simulink model "cps_fast_network_v2"  (R2012b)
settings: Solver=FixedStepDiscrete  StartTime=0.0  StopTime=8.5  RelTol=20e-5
model workspace (MAT data in the model file):
  ini_block_hpos = -0.4
  ini_block_vpos = 0.11
  ini_nozzle_vpos = 0.3
settings Model: Creator=pmosterm  LastModifiedBy=pmosterm
settings SolverCC: ZcThreshold=2e-5  MaxConsecutiveZCs=20  EnableConcurrentExecution=on  ConcurrentTasks=on  ZeroCrossAlgorithm=Adaptive  SolverResetMethod=Robust
settings DataIOCC: SignalLoggingSaveFormat=ModelDataLogs
settings OptimizationCC: InlineParams=on
settings DebuggingCC: ReadBeforeWriteMsg=DisableAll  WriteAfterWriteMsg=DisableAll  WriteAfterReadMsg=DisableAll  AlgebraicLoopMsg=error  UnderspecifiedInitializationDetection=Simplified  FcnCallInpInsideContextMsg=EnableAllAsWarning  ModelReferenceExtraNoncontSigs=warning
settings ModelReferenceCC: ModelReferenceNumInstancesAllowed=Single
settings GRTTargetCC: CombineOutputUpdateFcns=off  GRTInterface=on
settings ConfigurationSet: Description=SimMechanics 2G

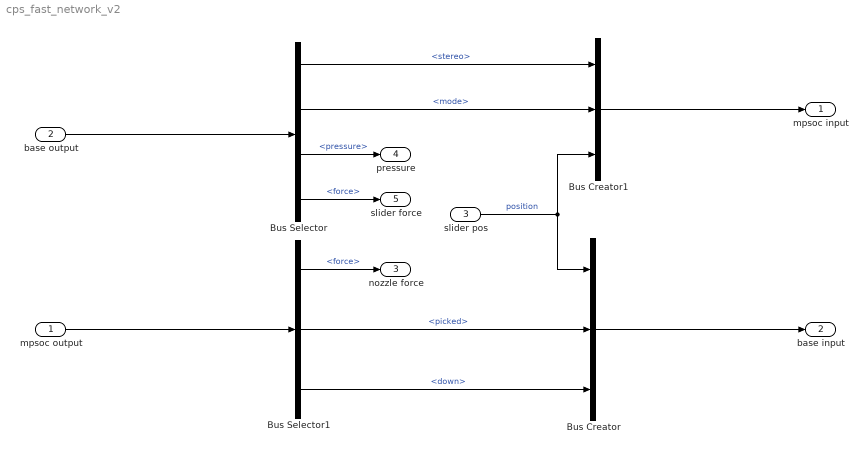
== system cps_fast_network_v2 ==
  mpsoc output : Inport  OutDataTypeStr=Bus: slBusNozzleControl
  base output : Inport  Port=2  OutDataTypeStr=Bus: slBusBaseOps
  slider pos : Inport  Port=3
  Bus Creator : BusCreator  Inputs=3
  Bus Creator1 : BusCreator  Inputs=3
  Bus Selector : BusSelector  OutputSignals=stereo,mode,pressure,force
  Bus Selector1 : BusSelector  OutputSignals=force,picked,down
  mpsoc input : Outport  OutDataTypeStr=Bus: slBusSliderControlOps  BusOutputAsStruct=on
  base input : Outport  Port=2  OutDataTypeStr=Bus: slBusSliderStatus  BusOutputAsStruct=on
  nozzle force : Outport  Port=3
  pressure : Outport  Port=4
  slider force : Outport  Port=5
  wires:
  Bus Selector/4 -> slider force/1  "<force>"
  Bus Selector1/1 -> nozzle force/1  "<force>"
  Bus Selector/2 -> Bus Creator1/2  "<mode>"
  Bus Selector/3 -> pressure/1  "<pressure>"
  Bus Selector1/2 -> Bus Creator/2  "<picked>"
  Bus Selector/1 -> Bus Creator1/1  "<stereo>"
  Bus Selector1/3 -> Bus Creator/3  "<down>"
  mpsoc output/1 -> Bus Selector1/1
  Bus Creator/1 -> base input/1
  base output/1 -> Bus Selector/1
  Bus Creator1/1 -> mpsoc input/1
  slider pos/1 -> Bus Creator1/3, Bus Creator/1  "position"
